simulink model "env_mdl_test"  (R2020b)
settings: Solver=VariableStepAuto  StartTime=0.0  StopTime=10.0  RelTol=1e-3
settings Model: Creator=brian  LastModifiedBy=brian

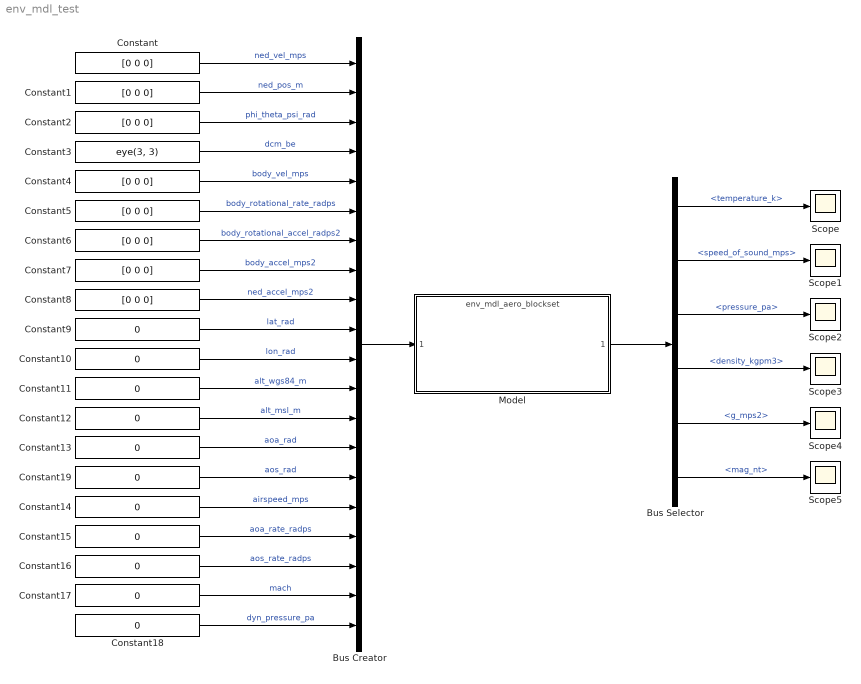
== system env_mdl_test ==
  Bus Creator : BusCreator  Inputs=20  OutDataTypeStr=Bus: VehicleState  NonVirtualBus=on
      settings: InheritFromInputs=off
  Bus Selector : BusSelector  OutputSignals=temperature_k,speed_of_sound_mps,pressure_pa,density_kgpm3,g_mps2,mag_nt
  Constant{,1..2,4..8} (8 alike) : Constant  Value=[0 0 0]
  Constant{9..19} (11 alike) : Constant  Value=0
  Constant3 : Constant  Value=eye(3, 3)
  Model : ModelReference  ModelNameDialog=env_mdl_aero_blockset.slx  SimulationMode=Normal  ModelReferenceVersion=1.1
  Scope{,1..5} (6 alike) : Scope
  wires:
  Bus Creator/1 -> Model/1
  Constant/1 -> Bus Creator/1  "ned_vel_mps"
  Constant1/1 -> Bus Creator/2  "ned_pos_m"
  Constant2/1 -> Bus Creator/3  "phi_theta_psi_rad"
  Constant3/1 -> Bus Creator/4  "dcm_be"
  Constant4/1 -> Bus Creator/5  "body_vel_mps"
  Constant5/1 -> Bus Creator/6  "body_rotational_rate_radps"
  Constant6/1 -> Bus Creator/7  "body_rotational_accel_radps2"
  Constant7/1 -> Bus Creator/8  "body_accel_mps2"
  Constant8/1 -> Bus Creator/9  "ned_accel_mps2"
  Constant9/1 -> Bus Creator/10  "lat_rad"
  Constant10/1 -> Bus Creator/11  "lon_rad"
  Constant11/1 -> Bus Creator/12  "alt_wgs84_m"
  Constant12/1 -> Bus Creator/13  "alt_msl_m"
  Constant13/1 -> Bus Creator/14  "aoa_rad"
  Constant14/1 -> Bus Creator/16  "airspeed_mps"
  Constant15/1 -> Bus Creator/17  "aoa_rate_radps"
  Constant16/1 -> Bus Creator/18  "aos_rate_radps"
  Constant17/1 -> Bus Creator/19  "mach"
  Constant18/1 -> Bus Creator/20  "dyn_pressure_pa"
  Model/1 -> Bus Selector/1
  Constant19/1 -> Bus Creator/15  "aos_rad"
  Bus Selector/1 -> Scope/1  "<temperature_k>"
  Bus Selector/2 -> Scope1/1  "<speed_of_sound_mps>"
  Bus Selector/3 -> Scope2/1  "<pressure_pa>"
  Bus Selector/4 -> Scope3/1  "<density_kgpm3>"
  Bus Selector/5 -> Scope4/1  "<g_mps2>"
  Bus Selector/6 -> Scope5/1  "<mag_nt>"
